simulink model "flightControlSystem"  (R2024a)
settings: Solver=ode3  StartTime=0  StopTime=TFinal  FixedStep=Ts  RelTol=1e-3  EnableMultiTasking=on
undefined symbols (not defined in the file): codertarget, Controller, DiscIntNeverNeededParam, Discrete, Estimator, g, init, orient_ref, pos_ref, Sensors, Time, Ts, var_acc_angle_N, var_bias_gyr_N, var_gyro_p_N, Vehicle
libraries: simulink x125, slpidlib x35, ctrlSharedLib x12, sharedtransform x10, eeGeneralControl x8, parrotlib x6, shareduavrstlib x1, simulink_need_slupdate x1
(part 11 of 11)

== matlab function flightControlSystem/Image Processing System/Vision Based Tracking ==
  data: in input; ang output; b output; x_new output; y_new output; sum_pixels output; sum_pix2 output; centroid_dist output
function [ang, b, x_new, y_new,sum_pixels,sum_pix2,centroid_dist] = calculate_ang(in)
    ang = 0;
    % b = ixbinarize(in);
 b=in;
 

    input = b;
    N = 1;
    out = zeros(2, N);
    x00 = zeros(1, N);
    x01 = zeros(1, N);
    x10 = zeros(1, N);
    
    [r, c] = size(input);
    
    for row = 1:r
        for col = 1:c
            if input(row, col) ~= 0 % on object pixel
               x10(input(row, col)) = row * 1 + x10(input(row, col)); 
               x01(input(row, col)) = col * 1 + x01(input(row, col));
               x00(input(row, col)) = x00(input(row, col)) + 1;
            end
        end
    end

    for i = 1:N
        if x00(i) ~= 0  % Check if x00 is not zero to avoid division by zero
            out(2, i) = x10(i) / x00(i);
            out(1, i) = x01(i) / x00(i);
        else
            out(2, i) = 0; % Assign default value when x00 is zero
            out(1, i) = 0; % Assign default value when x00 is zero
        end
    end
    
    x_new = out(1, 1)
    y_new = out(2, 1)

%      if x_new > 0.1   % Check if x_new is not zero to avoid division by zero
%          x_new = x_new+2
%       
%      elseif x_new<-0.1
%         x_new = x_new-2;
%      else
%          x_new=x_new
%          xe=x_new% Assign default angle when x_new is zero
%      end
%  
%      if y_new >0.1  % Check if x_new is not zero to avoid division by zero
%          y_new = y_new+2
% 
%       
%      elseif y_new<-0.1
%          y_new = y_new-2;
%      else
%          y_new=y_new
%          ye=y_new% Assign default angle when x_new is zero
%      end
%     
    if x_new ~= 0   % Check if x_new is not zero to avoid division by zero
        x_new = x_new - 80
        y_new = 60 - y_new
        ang = rad2deg(atan(y_new / x_new))
    else
        ang = 0; % Assign default angle when x_new is zero
    end
    mid_area1=b(55:65,75:85);
    centroid_dist = sqrt((x_new)^2 + (y_new)^2)
    area2=b(20:100,40:120);
  
    sum_pix2=sum(area2(:))
    sum_pixels=sum(mid_area1(:))
end

== matlab function flightControlSystem/Control System/Controller/Position Controller/Subsystem/MATLAB Function ==
  data: ddx input; ddy input; ddx_temp output; ddz input; ddy_temp output; ddz_temp output
function [ddx_temp, ddy_temp, ddz_temp] = fcn(ddx, ddy, ddz)
    persistent filterInitialized b a;
    noise_margin = 0.005; % Define the margin around zero to be considered as noise
    
    if isempty(filterInitialized)
        % Design the filter according to your specifications
        % Example: 2nd-order Butterworth low-pass filter with a cutoff frequency of 5 Hz and a sample rate of 100 Hz
        
        [b, a] = butter(2, (5/(100/2)), 'low');
        filterInitialized = true;
    end
    
    % Apply the filter to each acceleration component
    ddx_temp = filter(b, a, ddx);
    ddy_temp = filter(b, a, ddy);
    ddz_temp = filter(b, a, ddz);

    % Apply the bias correction (deadzone)
%     ddx_filtered = applyDeadzone(ddx_temp, noise_margin);
%     ddy_filtered = applyDeadzone(ddy_temp, noise_margin);
%     ddz_filtered = applyDeadzone(ddz_temp, noise_margin);
end

% function val_filtered = applyDeadzone(val, margin)
%     % Ensure that the function outputs the same type as the input
% %     if abs(val) < margin
%         val_filtered = cast(0, 'like', val); % Cast zero to the type of val
%     else
%         val_filtered = val;
%     end
% end
